simulink model "ex_6_1_sim"  (R2021a)
settings: Solver=FixedStepAuto  StartTime=0.0  StopTime=100  FixedStep=1  RelTol=1e-3
undefined symbols (not defined in the file): a, b, r1, s0, s1, w, zeta
settings Model: Creator=dbnun  LastModifiedBy=dimit

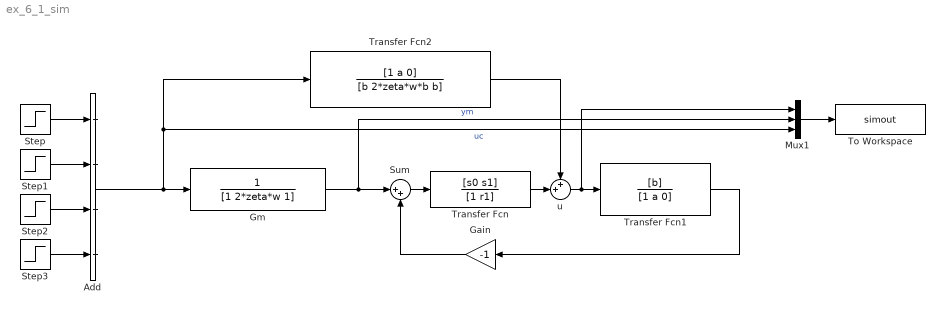
== system ex_6_1_sim ==
  Add : Sum  Inputs=++++
  Gain : Gain  Gain=-1
  Gm : TransferFcn  Denominator=[1 2*zeta*w 1]
  Mux1 : Mux  Inputs=3
  Step : Step  Time=0  SampleTime=0
  Step1 : Step  Time=25  After=-2  SampleTime=0
  Step2 : Step  Time=50  After=2  SampleTime=0
  Step3 : Step  Time=75  After=-2  SampleTime=0
  Sum : Sum  Inputs=|++
  To Workspace : ToWorkspace  VariableName=simout  SaveFormat=Timeseries  SampleTime=-1
  Transfer Fcn : TransferFcn  Numerator=[s0 s1]  Denominator=[1 r1]
  Transfer Fcn1 : TransferFcn  Numerator=[b]  Denominator=[1 a 0]
  Transfer Fcn2 : TransferFcn  Numerator=[1 a 0]  Denominator=[b 2*zeta*w*b b]
  u : Sum  Inputs=++|
  wires:
  Step/1 -> Add/1
  Step1/1 -> Add/2
  Step2/1 -> Add/3
  Step3/1 -> Add/4
  Add/1 -> Mux1/3, Transfer Fcn2/1, Gm/1  "uc"
  Gm/1 -> Sum/1, Mux1/2  "ym"
  Sum/1 -> Transfer Fcn/1
  Transfer Fcn/1 -> u/2
  Gain/1 -> Sum/2
  Transfer Fcn1/1 -> Gain/1
  Transfer Fcn2/1 -> u/1
  Mux1/1 -> To Workspace/1
  u/1 -> Mux1/1, Transfer Fcn1/1
